simulink model "PIDsim"  (R2018b)
settings: Solver=VariableStepAuto  StartTime=0.0  StopTime=70  RelTol=1e-3
values from neighbouring files (symbols this model uses):
  C = (pi*(100*10^-3)^2)/4    (= 0.00785398163397)    [Siviseviyesistemkodu.m]
  h = 0.225    [Siviseviyesistemkodu.m]
  P = 7.08    [Siviseviyesistemkodu.m]
  qin = 0.000087083333    (= 8.7083333e-05)    [Siviseviyesistemkodu.m]
  R = (h)/qo    [Siviseviyesistemkodu.m]
  td = 0.56    [Siviseviyesistemkodu.m]
  ti = 2.25    [Siviseviyesistemkodu.m]
settings Model: Creator=Yasin  LastModifiedBy=Yasin

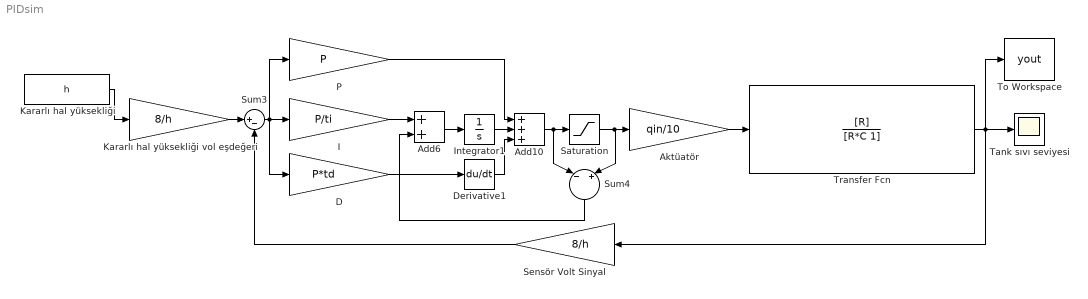
== system PIDsim ==
  Add10 : Sum  Inputs=+++
  Add6 : Sum
  Aktüatör : Gain  Gain=qin/10
  D : Gain  Gain=P*td
  Derivative1 : Derivative
  I : Gain  Gain=P/ti
  Integrator1 : Integrator
  "Kararlı hal yüksekliği " : Constant  Value=h
  Kararlı hal yüksekliği vol eşdeğeri : Gain  Gain=8/h
  P : Gain  Gain=P
  Saturation : Saturate  UpperLimit=10  LowerLimit=0  ZeroCross=off
  Sensör Volt Sinyal : Gain  Gain=8/h
  Sum3 : Sum  Inputs=|+-
  Sum4 : Sum  Inputs=|-|+|
  Tank sıvı seviyesi : Scope
  To Workspace : ToWorkspace  VariableName=yout  SaveFormat=Structure With Time  SampleTime=-1
      settings: Save2DSignal=2-D array (concatenate along first dimension)
  Transfer Fcn : TransferFcn  Numerator=[R]  Denominator=[R*C 1]
  wires:
  Sum4/1 -> Add6/2
  Add6/1 -> Integrator1/1
  Sensör Volt Sinyal/1 -> Sum3/2
  P/1 -> Add10/1
  Aktüatör/1 -> Transfer Fcn/1
  Add10/1 -> Saturation/1, Sum4/1
  Integrator1/1 -> Add10/2
  Kararlı hal yüksekliği vol eşdeğeri/1 -> Sum3/1
  Derivative1/1 -> Add10/3
  Sum3/1 -> D/1, P/1, I/1
  I/1 -> Add6/1
  D/1 -> Derivative1/1
  Transfer Fcn/1 -> To Workspace/1, Tank sıvı seviyesi/1, Sensör Volt Sinyal/1
  Saturation/1 -> Sum4/2, Aktüatör/1
  "Kararlı hal yüksekliği "/1 -> Kararlı hal yüksekliği vol eşdeğeri/1
